simulink model "heart_model_boolean"  (R2015a)
settings: Solver=ode3  StartTime=0.0  StopTime=size(sasignal,1)  FixedStep=1  RelTol=1e-6  AbsTol=1e-6
values from neighbouring files (symbols this model uses):
  beta1 = [-1 -0.3 -0.09 -0.3 -0.3 -0.3 -0.3 -0.3 -0.3 -0.3 -0.3 -0.3 ... (33 elements, 1x33)]    [pacemaker_heart_params.mat]
  beta3 = [200 200 200 200 200 200 200 200 200 200 200 200 ... (33 elements, 1x33)]    [pacemaker_heart_params.mat]
  beta4 = [-0.05 -0.05 -0.02 -0.02 -0.02 -0.02 -0.02 -0.02 -0.02 -0.02 -0.02 -0.02 ... (33 elements, 1x33)]    [pacemaker_heart_params.mat]
  delay = [15.5648 23.2106666667 5.18826666667 12.0149333333 12.8341333333 10.9226666667 18.5685333333 9.55733333333 12.8341333333 4.36906666667 5.46133333333 9.8304 ... (34 elements, 1x34)]    [pacemaker_heart_params.mat]
  gain = [0.1 0.1 0.1 0.1 0.07 0.1 0.1 0.1 0.1 0.1 0.1 0.1 ... (33 elements, 1x33)]    [pacemaker_heart_params.mat]
libraries: simulink x40, dspsrcs4 x1
(part 5 of 5)

== stateflow chart heart_model_boolean/Heart Model/VENTRICLE/SEP_LV (27)/Event generator ==
  settings: sampleTime=inf
  state state
  (default) -> ? [order 1]
  (default) -> state [order 1]
  state -> state [order 3] : [v>=138]/
      | event3;
  state -> state [order 1] : [v<20]/event1;
  state -> state [order 2] : [v>=20&&v<138]/event2;
  data: v input double =0
  events: event1 output EITHER_EDGE_EVENT; event2 output EITHER_EDGE_EVENT; event3 output EITHER_EDGE_EVENT

== stateflow chart heart_model_boolean/Heart Model/VENTRICLE/SEP_LV (27)/Hybrid set ==
  settings: sampleTime=inf
  state resting/
    entry:q=1;
  state stimulated/
    entry:q=2;
  state plateau/
    entry:q=4;
    vno=vn;
  state upstroke/
    entry:q=3;
  (default) -> ? [order 1]
  stimulated -> resting [order 2] : endpstim/vreset=v;reset;
  (default) -> resting [order 1]
  resting -> stimulated [order 1] : pstim/vreset=v;
      | vn=v;reset;
  resting -> upstroke [order 2] : event2/
      | vreset=v;reset;
  stimulated -> upstroke [order 1] : event2/
      | vreset=v;reset;
  plateau -> resting : event1/
      | vreset=v;reset;
  upstroke -> plateau : event3/
      | vreset=v;reset;
  data: q output double size=1 [1..4] =1; vreset output double =0; v input double size=1; vn local double =0; vno output double =0
  events: event1 input EITHER_EDGE_EVENT; reset output EITHER_EDGE_EVENT; event2 input EITHER_EDGE_EVENT; event3 input EITHER_EDGE_EVENT; pstim input RISING_EDGE_EVENT; endpstim input FALLING_EDGE_EVENT

== stateflow chart heart_model_boolean/Heart Model/VENTRICLE/SEP_LV_m (26)/Event generator ==
  settings: sampleTime=inf
  state state
  (default) -> ? [order 1]
  (default) -> state [order 1]
  state -> state [order 3] : [v>=138]/
      | event3;
  state -> state [order 1] : [v<20]/event1;
  state -> state [order 2] : [v>=20&&v<138]/event2;
  data: v input double =0
  events: event1 output EITHER_EDGE_EVENT; event2 output EITHER_EDGE_EVENT; event3 output EITHER_EDGE_EVENT

== stateflow chart heart_model_boolean/Heart Model/VENTRICLE/SEP_LV_m (26)/Hybrid set ==
  settings: sampleTime=inf
  state resting/
    entry:q=1;
  state stimulated/
    entry:q=2;
  state plateau/
    entry:q=4;
    vno=vn;
  state upstroke/
    entry:q=3;
  (default) -> ? [order 1]
  stimulated -> resting [order 2] : endpstim/vreset=v;reset;
  (default) -> resting [order 1]
  resting -> stimulated [order 1] : pstim/vreset=v;
      | vn=v;reset;
  resting -> upstroke [order 2] : event2/
      | vreset=v;reset;
  stimulated -> upstroke [order 1] : event2/
      | vreset=v;reset;
  plateau -> resting : event1/
      | vreset=v;reset;
  upstroke -> plateau : event3/
      | vreset=v;reset;
  data: q output double size=1 [1..4] =1; vreset output double =0; v input double size=1; vn local double =0; vno output double =0
  events: event1 input EITHER_EDGE_EVENT; reset output EITHER_EDGE_EVENT; event2 input EITHER_EDGE_EVENT; event3 input EITHER_EDGE_EVENT; pstim input RISING_EDGE_EVENT; endpstim input FALLING_EDGE_EVENT

== stateflow chart heart_model_boolean/Heart Model/VENTRICLE/SEP_RV (25)/Event generator ==
  settings: sampleTime=inf
  state state
  (default) -> ? [order 1]
  (default) -> state [order 1]
  state -> state [order 3] : [v>=138]/
      | event3;
  state -> state [order 1] : [v<20]/event1;
  state -> state [order 2] : [v>=20&&v<138]/event2;
  data: v input double =0
  events: event1 output EITHER_EDGE_EVENT; event2 output EITHER_EDGE_EVENT; event3 output EITHER_EDGE_EVENT

== stateflow chart heart_model_boolean/Heart Model/VENTRICLE/SEP_RV (25)/Hybrid set ==
  settings: sampleTime=inf
  state resting/
    entry:q=1;
  state stimulated/
    entry:q=2;
  state plateau/
    entry:q=4;
    vno=vn;
  state upstroke/
    entry:q=3;
  (default) -> ? [order 1]
  stimulated -> resting [order 2] : endpstim/vreset=v;reset;
  (default) -> resting [order 1]
  resting -> stimulated [order 1] : pstim/vreset=v;
      | vn=v;reset;
  resting -> upstroke [order 2] : event2/
      | vreset=v;reset;
  stimulated -> upstroke [order 1] : event2/
      | vreset=v;reset;
  plateau -> resting : event1/
      | vreset=v;reset;
  upstroke -> plateau : event3/
      | vreset=v;reset;
  data: q output double size=1 [1..4] =1; vreset output double =0; v input double size=1; vn local double =0; vno output double =0
  events: event1 input EITHER_EDGE_EVENT; reset output EITHER_EDGE_EVENT; event2 input EITHER_EDGE_EVENT; event3 input EITHER_EDGE_EVENT; pstim input RISING_EDGE_EVENT; endpstim input FALLING_EDGE_EVENT

== stateflow chart heart_model_boolean/Heart Model/VENTRICLE/SEP_RV_m (24)/Event generator ==
  settings: sampleTime=inf
  state state
  (default) -> ? [order 1]
  (default) -> state [order 1]
  state -> state [order 3] : [v>=138]/
      | event3;
  state -> state [order 1] : [v<20]/event1;
  state -> state [order 2] : [v>=20&&v<138]/event2;
  data: v input double =0
  events: event1 output EITHER_EDGE_EVENT; event2 output EITHER_EDGE_EVENT; event3 output EITHER_EDGE_EVENT

== stateflow chart heart_model_boolean/Heart Model/VENTRICLE/SEP_RV_m (24)/Hybrid set ==
  settings: sampleTime=inf
  state resting/
    entry:q=1;
  state stimulated/
    entry:q=2;
  state plateau/
    entry:q=4;
    vno=vn;
  state upstroke/
    entry:q=3;
  (default) -> ? [order 1]
  stimulated -> resting [order 2] : endpstim/vreset=v;reset;
  (default) -> resting [order 1]
  resting -> stimulated [order 1] : pstim/vreset=v;
      | vn=v;reset;
  resting -> upstroke [order 2] : event2/
      | vreset=v;reset;
  stimulated -> upstroke [order 1] : event2/
      | vreset=v;reset;
  plateau -> resting : event1/
      | vreset=v;reset;
  upstroke -> plateau : event3/
      | vreset=v;reset;
  data: q output double size=1 [1..4] =1; vreset output double =0; v input double size=1; vn local double =0; vno output double =0
  events: event1 input EITHER_EDGE_EVENT; reset output EITHER_EDGE_EVENT; event2 input EITHER_EDGE_EVENT; event3 input EITHER_EDGE_EVENT; pstim input RISING_EDGE_EVENT; endpstim input FALLING_EDGE_EVENT
